simulink model "Piezoelectric_Measurement_System"  (R2024a)
settings: Solver=VariableStepAuto  StartTime=0.0  StopTime=10.0  RelTol=1e-3
settings Model: Creator=javiercamacho  LastModifiedBy=javiercamacho

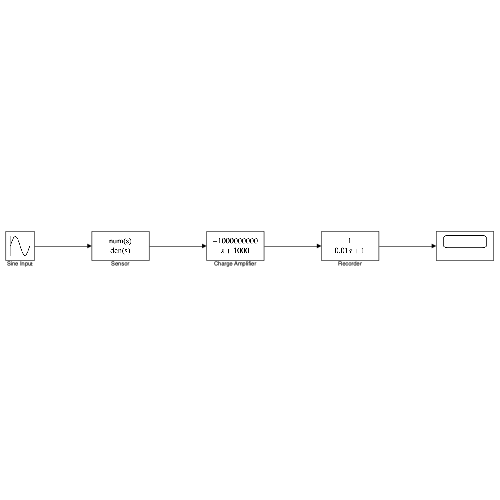
[thumbnail: Simulink's stored preview of the top-level diagram]
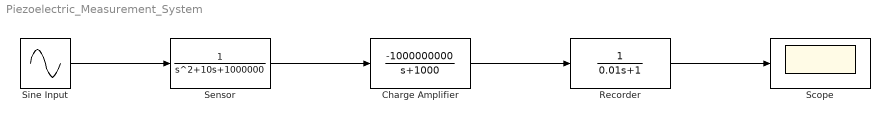
== system Piezoelectric_Measurement_System ==
  Charge Amplifier : TransferFcn  Numerator=[0 -1000000000]  Denominator=[1 1000]
  Recorder : TransferFcn  Numerator=[0 1]  Denominator=[0.01 1]
  Scope : Scope
  Sensor : TransferFcn  Numerator=[0 0 1]  Denominator=[1 10 1000000]
  Sine Input : Sin  Frequency=10  SampleTime=0
  wires:
  Sine Input/1 -> Sensor/1
  Sensor/1 -> Charge Amplifier/1
  Charge Amplifier/1 -> Recorder/1
  Recorder/1 -> Scope/1
